simulink model "secondModel"  (R2017a)
settings: Solver=VariableStepAuto  StartTime=0.0  StopTime=10.0  RelTol=1e-3
settings Model: Creator=bogdan.tamas  LastModifiedBy=bogdan.tamas

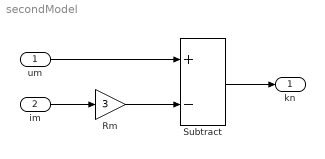
== system secondModel ==
  "um " : Inport
  im : Inport  Port=2
  Rm : Gain  Gain=3
  Subtract : Sum  Inputs=+-
  kn : Outport
  wires:
  im/1 -> Rm/1
  Rm/1 -> Subtract/2
  "um "/1 -> Subtract/1
  Subtract/1 -> kn/1
